simulink model "week1problem3_2019a"  (R2019a)
settings: Solver=VariableStepAuto  StartTime=0.0  StopTime=100  RelTol=1e-3
model workspace (MAT data in the model file):
  a1 = 0.01584
  b0 = 0.5792
  b1 = -0.5792
settings Model: Creator=rutvi  LastModifiedBy=rutvi

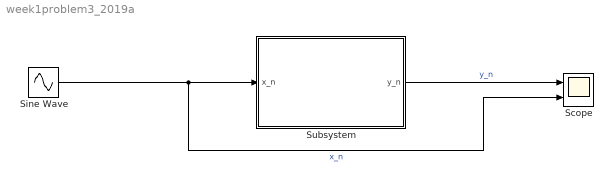
== system week1problem3_2019a ==
  Scope : Scope  NumInputPorts=2
  Sine Wave : Sin  Frequency=2*pi*100  Samples=5000  SampleTime=1/5000
  Subsystem : Subsystem
  wires:
  Sine Wave/1 -> Scope/2, Subsystem/1(x_n)  "x_n"
  Subsystem/1(y_n) -> Scope/1  "y_n"

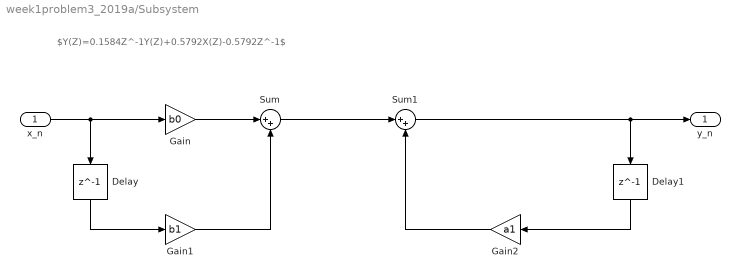
== system week1problem3_2019a/Subsystem ==
  note: $Y(Z)=0.1584Z^-1Y(Z)+0.5792X(Z)-0.5792Z^-1$
  x_n : Inport
  Delay : Delay  DelayLength=1
  Delay1 : Delay  DelayLength=1
  Gain : Gain  Gain=b0
  Gain1 : Gain  Gain=b1
  Gain2 : Gain  Gain=a1
  Sum : Sum  Inputs=|++
  Sum1 : Sum  Inputs=|++
  y_n : Outport
  wires:
  x_n/1 -> Gain/1, Delay/1
  Delay/1 -> Gain1/1
  Gain/1 -> Sum/1
  Gain1/1 -> Sum/2
  Sum/1 -> Sum1/1
  Sum1/1 -> Delay1/1, y_n/1
  Delay1/1 -> Gain2/1
  Gain2/1 -> Sum1/2
